simulink model "Simulink_recibir_datos"  (R2021a)
settings: Solver=VariableStepAuto  StartTime=0.0  StopTime=inf  RelTol=1e-3
libraries: instrumentseriallib x2
settings Model: Creator=Claudio  LastModifiedBy=rocio
settings DebuggingCC: UnderspecifiedInitializationDetection=Classic  MergeDetectMultiDrivingBlocksExec=none
settings ModelReferenceCC: PropagateSignalLabelsOutOfModel=off

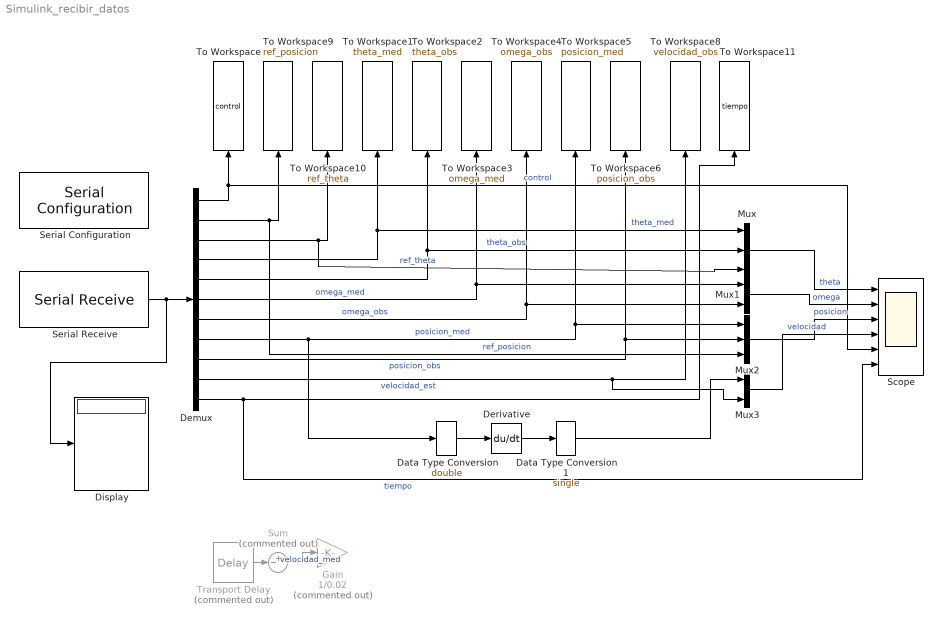
== system Simulink_recibir_datos ==
  Data Type Conversion : DataTypeConversion  OutDataTypeStr=double
  Data Type Conversion1 : DataTypeConversion  OutDataTypeStr=single
  Demux : Demux  Outputs=11
  Derivative : Derivative
  Display : Display
  Gain : Gain  Commented=on  Gain=1/0.02
  Mux : Mux  Inputs=3
  Mux1 : Mux  Inputs=2
  Mux2 : Mux  Inputs=3
  Mux3 : Mux  Inputs=2
  Scope : Scope  NumInputPorts=6
  Serial Configuration : instrumentseriallib/Serial Configuration  Priority=-200000  Port=COM3  ComPort=COM3  BaudRate=115200  DataBits=8  Parity=none  StopBits=1  ByteOrder=big-endian  FlowControl=none  Timeout=10  SimulateUsing=Interpreted execution  BlockInModel=on
  Serial Receive : instrumentseriallib/Serial Receive  Priority=1  Port=COM3  ComPort=COM3  DataType=single  SaveDataType=uint8  ToggleHeader=on  Header="[ 97   98   99  100 ]"  ToggleTerminator=off  Terminator=<none>  CustomTerminator=[]  ToggleDataSize=on  DataSize=[11 1]  EnableBlockingMode=on  ActionDataUnavailable=Output last received value  ActionWhenDataUnavailable=Output last received value  CustomValue=0  SampleTime=0.02  SimulateUsing=Interpreted execution  BlockInModel=on
  Sum : Sum  Commented=on  Inputs=+-|
  To Workspace : ToWorkspace  VariableName=control  SampleTime=-1
      settings: Save2DSignal=2-D array (concatenate along first dimension)
  To Workspace1 : ToWorkspace  VariableName=theta_med  SampleTime=-1
      settings: Save2DSignal=2-D array (concatenate along first dimension)
  To Workspace10 : ToWorkspace  VariableName=ref_theta  SampleTime=-1
      settings: Save2DSignal=2-D array (concatenate along first dimension)
  To Workspace11 : ToWorkspace  VariableName=tiempo  SampleTime=-1
      settings: Save2DSignal=2-D array (concatenate along first dimension)
  To Workspace2 : ToWorkspace  VariableName=theta_obs  SampleTime=-1
      settings: Save2DSignal=2-D array (concatenate along first dimension)
  To Workspace3 : ToWorkspace  VariableName=omega_med  SampleTime=-1
      settings: Save2DSignal=2-D array (concatenate along first dimension)
  To Workspace4 : ToWorkspace  VariableName=omega_obs  SampleTime=-1
      settings: Save2DSignal=2-D array (concatenate along first dimension)
  To Workspace5 : ToWorkspace  VariableName=posicion_med  SampleTime=-1
      settings: Save2DSignal=2-D array (concatenate along first dimension)
  To Workspace6 : ToWorkspace  VariableName=posicion_obs  SampleTime=-1
      settings: Save2DSignal=2-D array (concatenate along first dimension)
  To Workspace8 : ToWorkspace  VariableName=velocidad_obs  SampleTime=-1
      settings: Save2DSignal=2-D array (concatenate along first dimension)
  To Workspace9 : ToWorkspace  VariableName=ref_posicion  SampleTime=-1
      settings: Save2DSignal=2-D array (concatenate along first dimension)
  Transport Delay : TransportDelay  Commented=on  DelayTime=0.02
  wires:
  Serial Receive/1 -> Display/1, Demux/1
  Mux/1 -> Scope/1  "theta"
  Mux1/1 -> Scope/2  "omega"
  Mux2/1 -> Scope/3  "posicion"
  Mux3/1 -> Scope/4  "velocidad"
  Transport Delay/1 -> Sum/2
  Sum/1 -> Gain/1  "velocidad_med"
  Data Type Conversion/1 -> Derivative/1
  Derivative/1 -> Data Type Conversion1/1
  Demux/1 -> Scope/5, To Workspace/1  "control"
  Demux/2 -> Mux2/3, To Workspace9/1  "ref_posicion"
  Demux/3 -> Mux/3, To Workspace10/1  "ref_theta"
  Demux/4 -> To Workspace1/1, Mux/1  "theta_med"
  Demux/5 -> Mux/2, To Workspace2/1  "theta_obs"
  Demux/6 -> Mux1/1, To Workspace3/1  "omega_med"
  Demux/7 -> Mux1/2, To Workspace4/1  "omega_obs"
  Demux/8 -> Data Type Conversion/1, Mux2/1, To Workspace5/1  "posicion_med"
  Demux/9 -> Mux2/2, To Workspace6/1  "posicion_obs"
  Demux/10 -> Mux3/2, To Workspace8/1  "velocidad_est"
  Demux/11 -> Scope/6, To Workspace11/1  "tiempo"
  Data Type Conversion1/1 -> Mux3/1
